simulink model "daolibaixt4"  (Simulink 7.9)
settings: Solver=ode45  StartTime=0.0  StopTime=200  RelTol=1e-3
libraries: fuzblock x3
settings Model: Creator=fangzhen  LastModifiedBy=fangzhen
settings SolverCC: ZeroCrossControl=DisableAll

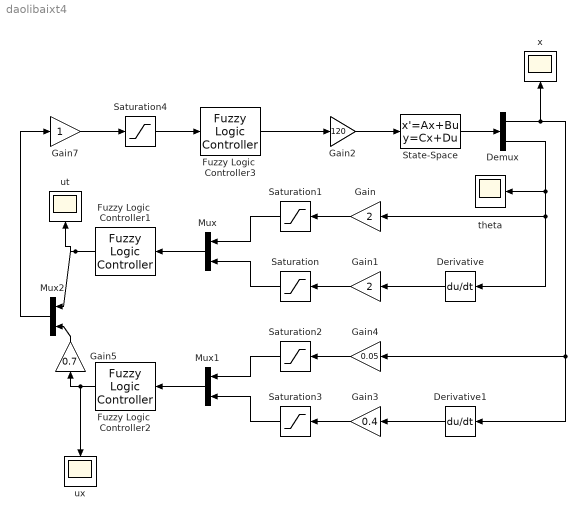
== system daolibaixt4 ==
  Demux : Demux  Outputs=2
  Derivative : Derivative
  Derivative1 : Derivative
  Fuzzy Logic  Controller1 : fuzblock/Fuzzy Logic  Controller  fis=daolibait
  Fuzzy Logic  Controller2 : fuzblock/Fuzzy Logic  Controller  fis=daolibaix
  Fuzzy Logic  Controller3 : fuzblock/Fuzzy Logic  Controller  fis=daolibai3_2
  Gain : Gain  Gain=2
  Gain1 : Gain  Gain=2
  Gain2 : Gain  Gain=120
  Gain3 : Gain  Gain=0.4  SampleTime=2
  Gain4 : Gain  Gain=0.05
  Gain5 : Gain  Gain=0.7
  Gain7 : Gain
  Mux : Mux  Inputs=2
  Mux1 : Mux  Inputs=2
  Mux2 : Mux  Inputs=2
  Saturation{,1..3} (4 alike) : Saturate  UpperLimit=2  LowerLimit=-2
  Saturation4 : Saturate  UpperLimit=3  LowerLimit=-3
  State-Space : StateSpace  A=[0,1,0,0; 0,0,10/12,0;0,0,0,1;0,0,100/12,0]  B=[0;1/9;0;1/12]  C=[1,0,0,0;0,0,1,0]  D=[0;0]  X0=[20;-4;-0.1;-0.10]  ContinuousStateAttributes='rad'
  theta : Scope
      settings: YMin=-60  YMax=50
  ut : Scope
      settings: YMin=-60  YMax=50  SaveName=ScopeData3
  ux : Scope
      settings: YMin=-60  YMax=50  SaveName=ScopeData2
  x : Scope
      settings: TimeRange=200  YMin=-15  YMax=20
  wires:
  Gain2/1 -> State-Space/1
  Demux/1 -> Gain4/1, Derivative1/1, x/1
  Derivative1/1 -> Gain3/1
  State-Space/1 -> Demux/1
  Gain4/1 -> Saturation2/1
  Gain3/1 -> Saturation3/1
  Demux/2 -> Derivative/1, Gain/1, theta/1
  Derivative/1 -> Gain1/1
  Gain1/1 -> Saturation/1
  Gain/1 -> Saturation1/1
  Fuzzy Logic  Controller3/1 -> Gain2/1
  Saturation4/1 -> Fuzzy Logic  Controller3/1
  Gain7/1 -> Saturation4/1
  Saturation1/1 -> Mux/1
  Saturation/1 -> Mux/2
  Mux/1 -> Fuzzy Logic  Controller1/1
  Saturation3/1 -> Mux1/2
  Mux1/1 -> Fuzzy Logic  Controller2/1
  Fuzzy Logic  Controller1/1 -> Mux2/1, ut/1
  Fuzzy Logic  Controller2/1 -> ux/1, Gain5/1
  Mux2/1 -> Gain7/1
  Saturation2/1 -> Mux1/1
  Gain5/1 -> Mux2/2
